simulink model "pendulum_3rdgen"  (R2017a)
settings: Solver=VariableStepAuto  StartTime=0.0  StopTime=25  RelTol=1e-3
InitFcn:
  | L = 0.495;
  | m = 0.43;
  | d = 0.023;
  | J = (1/12)*(m*L*L+m*d*d);
  | g = 9.81;
  | c = 0.00135;
undefined symbols (not defined in the file): X, Y, Z
libraries: sm_lib x9, nesl_utility x4
settings Model: Creator=user  LastModifiedBy=nikhi

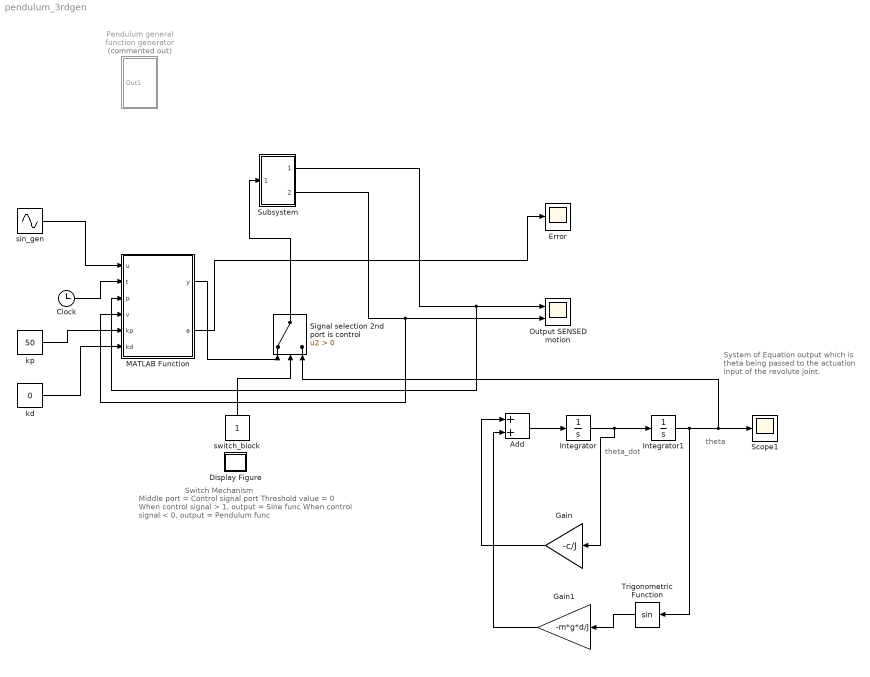
== system pendulum_3rdgen ==
  note: System of Equation output which is theta being passed to the
      | actuation input of the revolute joint.
  note: theta_dot
  note: theta
  note: Switch Mechanism
  note: Middle port = Control signal port
      | Threshold value = 0
      | When control signal > 1, output = Sine func
      | When control signal < 0, output = Pendulum func
  Add : Sum
  Clock : Clock
  Display Figure : Subsystem  Tag=Help  Description="Help callback for conveyor model: mech_conveyor.  Opens Help browser to Type 19 marker at documentation for this tutorial model."  mask(Help callback){}
      settings: OpenFcn=helpview([docroot '/toolbox/physmod/mech/mech.map'], 'mech_conveyor_help');
      mask Display: image(imread('info.bmp'))
  Error : Scope
  Gain : Gain  Gain=-c/J
  Gain1 : Gain  Gain=-m*g*d/J
  Integrator : Integrator
  Integrator1 : Integrator  InitialCondition=3.14/3
  MATLAB Function : MATLAB Function  TreatAsAtomicUnit=on
  Output SENSED motion : Scope  NumInputPorts=2
  Pendulum general function generator : Subsystem  Commented=on
  Scope1 : Scope
  Signal selection 2nd port is control : Switch  Criteria=u2 > Threshold
  Subsystem : Subsystem
  Trigonometric Function : Trigonometry
  kd : Constant  Value=0
  kp : Constant  Value=50
  sin_gen : Sin  SampleTime=0
      settings: AttributesFormatString=|
      | Amplitude = %<Amplitude>
      | Frequency = %<Frequency>
      | Phase = %<Phase>
      | %<SineType>
  switch_block : Constant
      settings: AttributesFormatString=Input value = %<Value>
  wires:
  switch_block/1 -> Signal selection 2nd port is control/2
  Integrator/1 -> Gain/1, Integrator1/1
  Add/1 -> Integrator/1
  Gain1/1 -> Add/2
  Integrator1/1 -> Signal selection 2nd port is control/3, Scope1/1, Trigonometric Function/1
  Gain/1 -> Add/1
  Trigonometric Function/1 -> Gain1/1
  Signal selection 2nd port is control/1 -> Subsystem/1(In1)
  Subsystem/1(Out1) -> MATLAB Function/3(p), Output SENSED motion/1
  Subsystem/2(Out2) -> MATLAB Function/4(v), Output SENSED motion/2
  MATLAB Function/1(y) -> Signal selection 2nd port is control/1
  sin_gen/1 -> MATLAB Function/1(u)
  Clock/1 -> MATLAB Function/2(t)
  kp/1 -> MATLAB Function/5(kp)
  kd/1 -> MATLAB Function/6(kd)
  MATLAB Function/2(e) -> Error/1

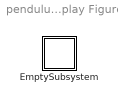
== system pendulum_3rdgen/Display Figure ==
  EmptySubsystem : Subsystem

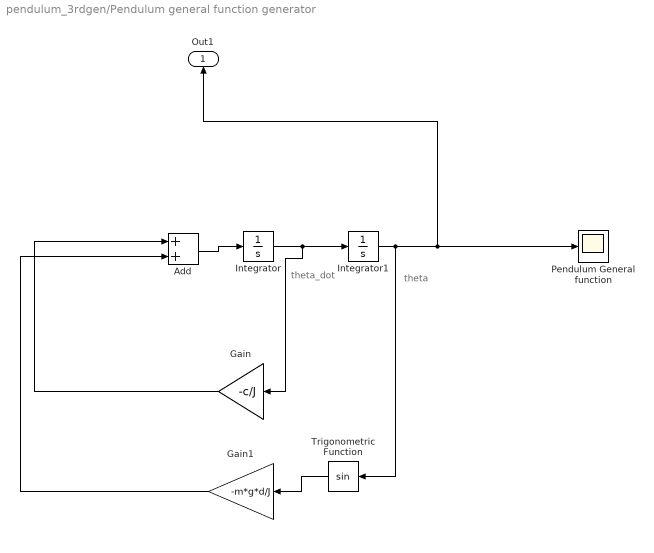
== system pendulum_3rdgen/Pendulum general function generator ==
  note: theta
  note: theta_dot
  Add : Sum
  Gain : Gain  Gain=-c/J
  Gain1 : Gain  Gain=-m*g*d/J
  Integrator : Integrator
  Integrator1 : Integrator  InitialCondition=3.14/3
  Pendulum General function : Scope
  Trigonometric Function : Trigonometry
  Out1 : Outport
  wires:
  Integrator1/1 -> Out1/1, Pendulum General function/1, Trigonometric Function/1
  Integrator/1 -> Gain/1, Integrator1/1
  Gain1/1 -> Add/2
  Gain/1 -> Add/1
  Add/1 -> Integrator/1
  Trigonometric Function/1 -> Gain1/1

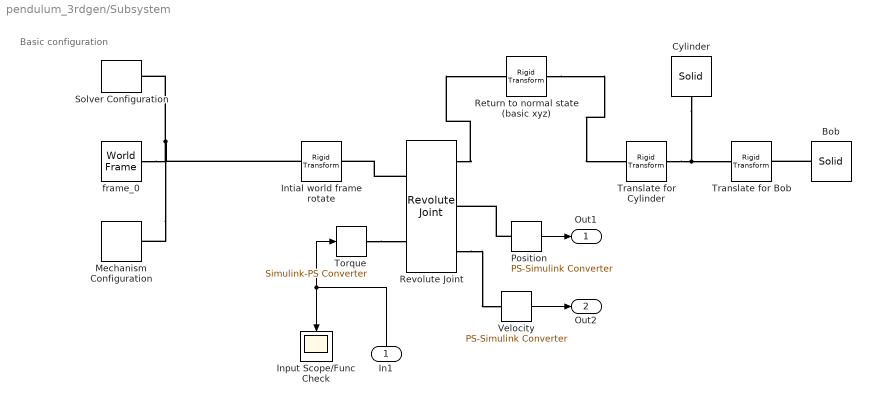
== system pendulum_3rdgen/Subsystem ==
  note: Basic configuration
  In1 : Inport
  " Cylinder" : sm_lib/Body Elements/Solid  InertiaType=CalculateFromGeometry  Mass=1  MassUnits=kg  CenterOfMass=[0 0 0]  CenterOfMassUnits=m  MomentsOfInertia=[1 1 1]  MomentsOfInertiaUnits=kg*m^2  ProductsOfInertia=[0 0 0]  ProductsOfInertiaUnits=kg*m^2  DensityBased=on  Density=1000  DensityUnits=kg/(m^3)  DoExposeReferenceFrame=on  SerializedFrames=<Frames/>  GraphicType=FromGeometry  MarkerShape=Sphere  MarkerSize=10  MarkerSizeUnits=m  GraphicVisPropType=SimpleVisualProperties  GraphicDiffuseColor=[0.2 0.0 1.0]  GraphicSpecularColor=[0.5 0.5 0.5 1.0]  GraphicAmbientColor=[0.15 0.15 0.15 1.0]  GraphicEmissiveColor=[0.0 0.0 0.0 1.0]  GraphicShininess=75  GraphicOpacity=1.0  GeometryShape=Cylinder  RectangleSize=[1 1]  RectangleSizeUnits=m  BrickDimensions=[5 5 5]  BrickDimensionUnits=cm  CylinderRadius=0.1  CylinderRadiusUnits=cm  CylinderLength=10  CylinderLengthUnits=cm  SphereRadius=0.5  SphereRadiusUnits=cm  EllipsoidRadii=[1 1 1]  EllipsoidRadiiUnits=m  ExtrusionCrossSection=[1 1; -1 1; -1 -1; 1 -1]  ExtrusionCrossSectionUnits=cm  ExtrusionLength=1  ExtrusionLengthUnits=m  PolygonNumSides=3  PolygonOuterRadius=1  PolygonOuterRadiusUnits=m  ExtGeomFileType=STL  ExtGeomFileUnits=m  RevolutionCrossSection=[1 1; 1 -1; 2 -1; 2 1]  RevolutionCrossSectionUnits=m  RevolutionExtent=Full  RevolutionAngle=180  RevolutionAngleUnits=deg
  Bob : sm_lib/Body Elements/Solid  InertiaType=CalculateFromGeometry  Mass=1  MassUnits=kg  CenterOfMass=[0 0 0]  CenterOfMassUnits=m  MomentsOfInertia=[1 1 1]  MomentsOfInertiaUnits=kg*m^2  ProductsOfInertia=[0 0 0]  ProductsOfInertiaUnits=kg*m^2  DensityBased=on  Density=1000  DensityUnits=kg/(m^3)  DoExposeReferenceFrame=on  SerializedFrames=<Frames/>  GraphicType=FromGeometry  MarkerShape=Sphere  MarkerSize=10  MarkerSizeUnits=m  GraphicVisPropType=SimpleVisualProperties  GraphicDiffuseColor=[1.0 0.0 0.0]  GraphicSpecularColor=[0.5 0.5 0.5 1.0]  GraphicAmbientColor=[0.15 0.15 0.15 1.0]  GraphicEmissiveColor=[0.0 0.0 0.0 1.0]  GraphicShininess=75  GraphicOpacity=1.0  GeometryShape=Sphere  RectangleSize=[1 1]  RectangleSizeUnits=m  BrickDimensions=[1 1 1]  BrickDimensionUnits=cm  CylinderRadius=1  CylinderRadiusUnits=m  CylinderLength=1  CylinderLengthUnits=m  SphereRadius=1  SphereRadiusUnits=cm  EllipsoidRadii=[1 1 1]  EllipsoidRadiiUnits=m  ExtrusionCrossSection=[1 1; -1 1; -1 -1; 1 -1]  ExtrusionCrossSectionUnits=m  ExtrusionLength=1  ExtrusionLengthUnits=m  PolygonNumSides=3  PolygonOuterRadius=1  PolygonOuterRadiusUnits=m  ExtGeomFileType=STL  ExtGeomFileUnits=m  RevolutionCrossSection=[1 1; 1 -1; 2 -1; 2 1]  RevolutionCrossSectionUnits=m  RevolutionExtent=Full  RevolutionAngle=180  RevolutionAngleUnits=deg
  Input Scope/Func Check : Scope
  Intial world frame rotate : sm_lib/Frames and Transforms/Rigid Transform  TranslationMethod=None  TranslationStandardOffset=5  TranslationLengthUnit=cm  TranslationStandardAxis=+Z  TranslationCartesianOffset=[0 0 0]  TranslationROffset=0  TranslationROffsetUnits=m  TranslationZOffset=0  TranslationZOffsetUnits=m  TranslationThetaOffset=0  TranslationThetaOffsetUnits=deg  RotationMethod=StandardAxis  RotationAngleUnits=deg  RotationStandardAxis=+X  RotationAngle=90  RotationArbitraryAxis=[0 0 1]  FollAlignAxisA=+X  BaseAlignAxisA=+Y  FollAlignAxisB=+Y  BaseAlignAxisB=+Z  RotationSequenceAxes=FollowerAxes  RotationSequence=XYX  RotationSequenceAngles=[0 0 0]  RotationSequenceAnglesUnits=deg  RotationMatrix=[1 0 0; 0 1 0; 0 0 1]
      settings: AttributesFormatString=|
      | %<RotationAngle>%<RotationAngleUnits>
      | about %<RotationStandardAxis>
  Mechanism Configuration : sm_lib/Utilities/Mechanism Configuration  UniformGravity=Constant  GravityVector=[0 0 -10]  GravityUnits=m/s^2  LinearizationDelta=0.001
      settings: AttributesFormatString=g = %<GravityVector>%<GravityUnits>
  Position : nesl_utility/PS-Simulink Converter  PhysicalDomain=network_engine_domain  SubClassName=ps_output  LeftPortType=input  RightPortType=output  PseudoPeriodic=off  Frequencies=[]  Unit=rad  AffineConversion=off
  Return to normal state (basic xyz) : sm_lib/Frames and Transforms/Rigid Transform  TranslationMethod=None  TranslationStandardOffset=5.5  TranslationLengthUnit=cm  TranslationStandardAxis=+Z  TranslationCartesianOffset=[0 0 0]  TranslationROffset=0  TranslationROffsetUnits=m  TranslationZOffset=0  TranslationZOffsetUnits=m  TranslationThetaOffset=0  TranslationThetaOffsetUnits=deg  RotationMethod=StandardAxis  RotationAngleUnits=deg  RotationStandardAxis=-X  RotationAngle=90  RotationArbitraryAxis=[1 1 1]  FollAlignAxisA=-Y  BaseAlignAxisA=+Z  FollAlignAxisB=+Z  BaseAlignAxisB=+Y  RotationSequenceAxes=BaseAxes  RotationSequence=ZYZ  RotationSequenceAngles=[0 0 0]  RotationSequenceAnglesUnits=deg  RotationMatrix=[1 0 0; 0 1 0; 0 0 1]
      settings: AttributesFormatString=|
      | %<RotationAngle>%<RotationAngleUnits>
      | about %<RotationStandardAxis>
  Revolute Joint : sm_lib/Joints/Revolute Joint  SenseConstraintForce=off  SenseConstraintForceX=off  SenseConstraintForceY=off  SenseConstraintForceZ=off  SenseConstraintTorque=off  SenseConstraintTorqueX=off  SenseConstraintTorqueY=off  SenseConstraintTorqueZ=off  SenseTotalForce=off  SenseTotalForceX=off  SenseTotalForceY=off  SenseTotalForceZ=off  SenseTotalTorque=off  SenseTotalTorqueX=off  SenseTotalTorqueY=off  SenseTotalTorqueZ=off  CompositeWrenchDir=FollowerOnBase  CompositeWrenchFrame=BaseFrame  EquilibriumPosition=0  EquilibriumPositionUnits=deg  SpringStiffness=0  SpringStiffnessUnits=N*m/deg  DampingCoefficient=0.1  DampingCoefficientUnits=N*m/(deg/s)  TorqueActuationMode=InputTorque  MotionActuationMode=ComputedMotion  SensePosition=on  SenseVelocity=on  SenseAcceleration=off  SenseTorqueForce=off  PositionTargetSpecify=on  PositionTargetPriority=High  PositionTargetValue=0  PositionTargetValueUnits=deg  VelocityTargetSpecify=off  VelocityTargetPriority=High  VelocityTargetValue=0  VelocityTargetValueUnits=deg/s
  Solver Configuration : nesl_utility/Solver Configuration  PhysicalDomain=network_engine_domain  SubClassName=solver  LeftPortType=input  RightPortType=generic  Accelerate=off  Tones=[]  Harmonics=[]  SimulateNoise=off  Profile=off  UseLocalSampling=off  EnableSwitchedLinearOptims=on  FrequencyDomain=off  UseCCode=off  RelTol=0.001  AbsTol=1e-06  MinStep=1e-09  ToWorkspace=off  RevertToSquareIcSolve=off  NumHomotopyIterations=100  PhasorMode=off  PhasorModeNumHarmonics=1  OverrideAbsTol=off  DoDC=off  ResidualTolerance=1e-09  UseLocalSolver=off  LocalSolverChoice=NE_BACKWARD_EULER_ADVANCER  LocalSolverSampleTime=0.001  DoFixedCost=off  MaxNonlinIter=3  MaxModeIter=2  LinearAlgebra=Sparse  DelaysMemoryBudget=1024  AutomaticFiltering=on  FilteringTimeConstant=0.001
  Torque : nesl_utility/Simulink-PS Converter  PhysicalDomain=network_engine_domain  SubClassName=ps_input  LeftPortType=input  RightPortType=output  PseudoPeriodic=off  Frequencies=[]  NoiseDistribution=none  NoiseParameters=[]  Unit=1  AffineConversion=off  FilteringAndDerivatives=zero  SimscapeFilterOrder=1  InputFilterTimeConstant=0.001  UdotUserProvided=1
  Translate for Bob : sm_lib/Frames and Transforms/Rigid Transform  TranslationMethod=StandardAxis  TranslationStandardOffset=5  TranslationLengthUnit=cm  TranslationStandardAxis=-Z  TranslationCartesianOffset=[0 0 0]  TranslationROffset=0  TranslationROffsetUnits=m  TranslationZOffset=0  TranslationZOffsetUnits=m  TranslationThetaOffset=0  TranslationThetaOffsetUnits=deg  RotationMethod=None  RotationAngleUnits=deg  RotationStandardAxis=-X  RotationAngle=90  RotationArbitraryAxis=[1 1 1]  FollAlignAxisA=-Y  BaseAlignAxisA=+Z  FollAlignAxisB=+Z  BaseAlignAxisB=+Y  RotationSequenceAxes=BaseAxes  RotationSequence=ZYZ  RotationSequenceAngles=[0 0 0]  RotationSequenceAnglesUnits=deg  RotationMatrix=[1 0 0; 0 1 0; 0 0 1]
      settings: AttributesFormatString=|
      | %<TranslationStandardOffset>cm
      | %<TranslationStandardAxis>
  Translate for Cylinder : sm_lib/Frames and Transforms/Rigid Transform  TranslationMethod=StandardAxis  TranslationStandardOffset=5  TranslationLengthUnit=cm  TranslationStandardAxis=-Z  TranslationCartesianOffset=[0 0 0]  TranslationROffset=0  TranslationROffsetUnits=m  TranslationZOffset=0  TranslationZOffsetUnits=m  TranslationThetaOffset=0  TranslationThetaOffsetUnits=deg  RotationMethod=None  RotationAngleUnits=deg  RotationStandardAxis=+X  RotationAngle=90  RotationArbitraryAxis=[0 0 1]  FollAlignAxisA=+X  BaseAlignAxisA=+Y  FollAlignAxisB=+Y  BaseAlignAxisB=+Z  RotationSequenceAxes=FollowerAxes  RotationSequence=XYX  RotationSequenceAngles=[0 0 0]  RotationSequenceAnglesUnits=deg  RotationMatrix=[1 0 0; 0 1 0; 0 0 1]
      settings: AttributesFormatString=|
      | %<TranslationStandardOffset>cm
      | %<TranslationStandardAxis>
  Velocity : nesl_utility/PS-Simulink Converter  PhysicalDomain=network_engine_domain  SubClassName=ps_output  LeftPortType=input  RightPortType=output  PseudoPeriodic=off  Frequencies=[]  Unit=rad/s  AffineConversion=off
  frame_0 : sm_lib/Frames and Transforms/World Frame
  Out1 : Outport
  Out2 : Outport  Port=2
  wires:
  Position/1 -> Out1/1
  In1/1 -> Torque/1, Input Scope/Func Check/1
  Velocity/1 -> Out2/1
  connections:
  Revolute Joint/LConn1 -- Intial world frame rotate/RConn1
  Position/LConn1 -- Revolute Joint/RConn2
  Revolute Joint/RConn1 -- Return to normal state (basic xyz)/LConn1
  " Cylinder"/RConn1 -- Translate for Cylinder/RConn1 -- Translate for Bob/LConn1
  Bob/RConn1 -- Translate for Bob/RConn1
  Torque/RConn1 -- Revolute Joint/LConn2
  Revolute Joint/RConn3 -- Velocity/LConn1
  Return to normal state (basic xyz)/RConn1 -- Translate for Cylinder/LConn1
  frame_0/RConn1 -- Mechanism Configuration/RConn1 -- Intial world frame rotate/LConn1 -- Solver Configuration/RConn1

== system pendulum_3rdgen/Display Figure/EmptySubsystem ==

== matlab function pendulum_3rdgen/MATLAB Function ==
  data: u input; y output; t input; p input; v input; kp input; kd input; e output
function [y, e]= fcn(u,t,p,v,kp,kd)
p_des = -pi/6; %desired position
%p_des = u;
v_des = 5*cos(t);
e = p - p_des; %error
y = -kp*e-kd*(v-v_des);
%y = u;  %-0.43*9.8*0.5/.009;
